simulink model "MPC_mobile_base_KIN_IPOPT_fast"  (R2018b)
settings: Solver=ode4  StartTime=0.0  StopTime=inf  FixedStep=Tsample  RelTol=1e-3
values from neighbouring files (symbols this model uses):
  initialize_starting_point = 1    [init_prova_vera1.mat]    (also in init_prova_vera3.mat; prova_vera1.mat = 0; prova_vera2.mat = 0)
  N = length(q)    [FK.m]    (also in FK_generation.m = size(DHTABLE,1); init_prova_vera1.mat = 10; init_prova_vera3.mat = 10; jacobian_MM.m)
  Np = 18    [init_prova_vera1.mat]    (also in init_prova_vera3.mat; initialization.m = Lf*2 + Lp*6; prova_vera1.mat; prova_vera2.mat)
  T = cell(N+1,1)    [FK.m]    (also in init_prova_vera1.mat = 0.5; init_prova_vera3.mat = 0.5; jacobian_MM.m; matlabultimo.mat = 0.5)
  Tsample = 0.01    [init_prova_vera1.mat]    (also in init_prova_vera3.mat; matlabultimo.mat; prova_vera1.mat; prova_vera2.mat)
  x0_val = [0 0 0 -5.2235 -1.0817 -2.0377 -0.3426 0.6332 1.3451 0.0238792670666 0.415141969475 1.22261425872 ... (18 elements, 18x1)]    [init_prova_vera1.mat]    (also in init_prova_vera3.mat; matlabultimo.mat = [0 0 0 2.943 -0.9502 1.3671 -2.8338 -2.9626 -0.0003 0.671714; prova_vera1.mat; prova_vera2.mat)
  xd = [0 0 0 0 0 0 0 0 0 0.0238792670666 0.415141969475 1.22261425872 ... (1458 elements, 18x81)]    [init_prova_vera1.mat]    (also in init_prova_vera3.mat; liveplot.m = evalin('base','xd'); matlabultimo.mat = [0 0 0 0 0 0 0 0 0 -0.528285242967 -0.106449885857 1.3372295; prova_vera1.mat)
undefined symbols (not defined in the file or in its folder): DiscIntNeverNeededParam
libraries: simulink x3
settings Model: Creator=francesco  LastModifiedBy=francesco
settings ModelReferenceCC: PropagateVarSize=Only when enabling

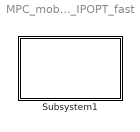
== system MPC_mobile_base_KIN_IPOPT_fast ==
  Subsystem1 : Subsystem  InitFcn=initialization

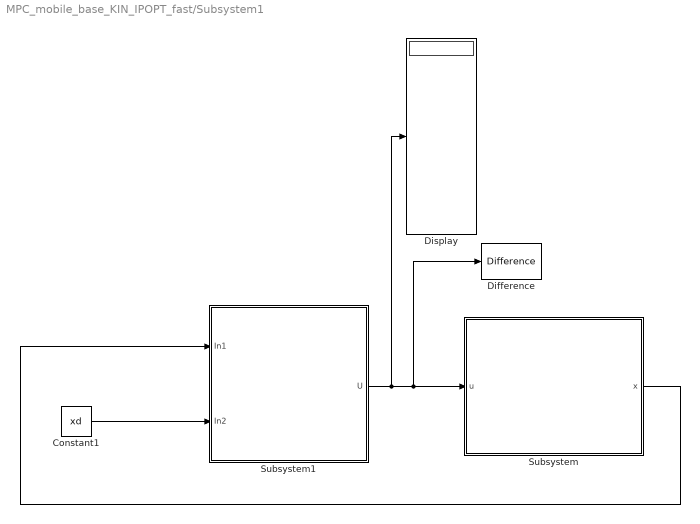
== system MPC_mobile_base_KIN_IPOPT_fast/Subsystem1 ==
  Constant1 : Constant  Value=xd
  Difference : simulink/Discrete/Difference  ICPrevInput=0.0  OutMin=[]  OutMax=[]  OutDataType=fixdt(1, 16)  OutScaling=2^-10  DoSatur=off
  Display : Display
  Subsystem : Subsystem
      mask Display: disp('{\bf\fontsize{10}KINEMATIC SYSTEM}', 'texmode','on');
  Subsystem1 : Subsystem
  wires:
  Subsystem1/1(U) -> Display/1, Difference/1, Subsystem/1(u)
  Constant1/1 -> Subsystem1/2(In2)
  Subsystem/1(x) -> Subsystem1/1(In1)

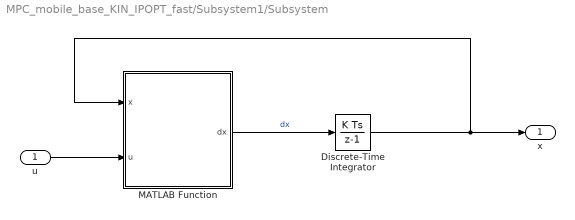
== system MPC_mobile_base_KIN_IPOPT_fast/Subsystem1/Subsystem ==
  u : Inport
  Discrete-Time Integrator : DiscreteIntegrator  InitialCondition=x0_val  SampleTime=Tsample  ICPrevOutput=DiscIntNeverNeededParam  ICPrevScaledInput=DiscIntNeverNeededParam
  MATLAB Function : MATLAB Function  TreatAsAtomicUnit=on
  x : Outport  SampleTime=Tsample
  wires:
  u/1 -> MATLAB Function/2(u)
  MATLAB Function/1(dx) -> Discrete-Time Integrator/1  "dx"
  Discrete-Time Integrator/1 -> MATLAB Function/1(x), x/1

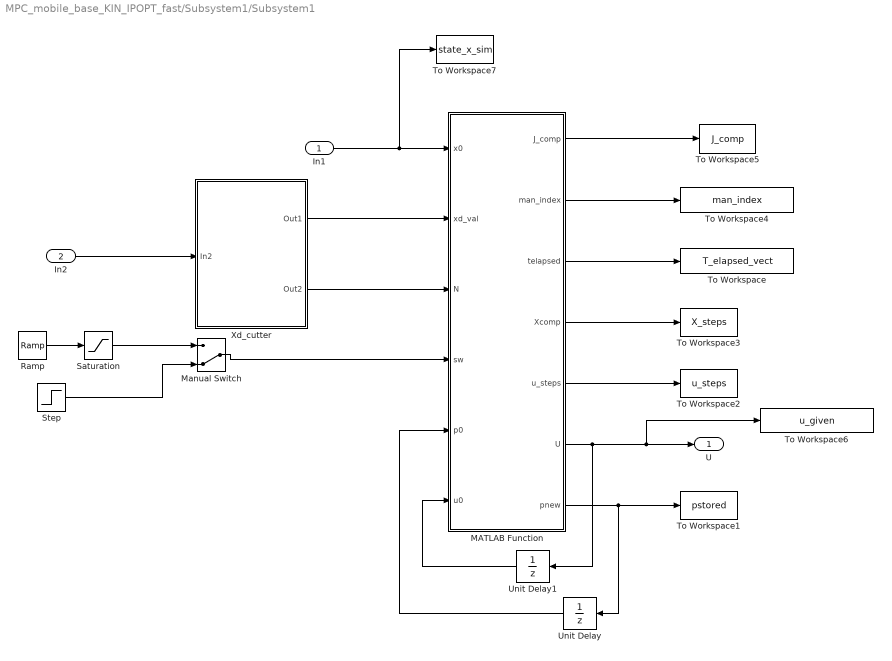
== system MPC_mobile_base_KIN_IPOPT_fast/Subsystem1/Subsystem1 ==
  In1 : Inport
  In2 : Inport  Port=2
  MATLAB Function : MATLAB Function  TreatAsAtomicUnit=on
  Manual Switch : ManualSwitch  CurrentSetting=0
  Ramp : simulink/Sources/Ramp  slope=1.5  start=15  InitialOutput=0
  Saturation : Saturate  UpperLimit=1
  Step : Step  Time=0  SampleTime=0
  To Workspace : ToWorkspace  VariableName=T_elapsed_vect  SampleTime=T
  To Workspace1 : ToWorkspace  VariableName=pstored  SampleTime=-1
  To Workspace2 : ToWorkspace  VariableName=u_steps  SaveFormat=Structure  SampleTime=-1
  To Workspace3 : ToWorkspace  VariableName=X_steps  SaveFormat=Structure  SampleTime=-1
  To Workspace4 : ToWorkspace  VariableName=man_index  SampleTime=T
  To Workspace5 : ToWorkspace  VariableName=J_comp  SampleTime=-1
  To Workspace6 : ToWorkspace  VariableName=u_given  SampleTime=T
  To Workspace7 : ToWorkspace  VariableName=state_x_sim  SampleTime=T
  Unit Delay : UnitDelay  InitialCondition=zeros(Np,1)  SampleTime=T
  Unit Delay1 : UnitDelay  InitialCondition=zeros(8,1)  SampleTime=T
  Xd_cutter : Subsystem
  U : Outport
  wires:
  MATLAB Function/7(pnew) -> To Workspace1/1, Unit Delay/1
  MATLAB Function/6(U) -> Unit Delay1/1, To Workspace6/1, U/1
  Unit Delay/1 -> MATLAB Function/5(p0)
  MATLAB Function/3(telapsed) -> To Workspace/1
  Unit Delay1/1 -> MATLAB Function/6(u0)
  MATLAB Function/5(u_steps) -> To Workspace2/1
  MATLAB Function/4(Xcomp) -> To Workspace3/1
  In2/1 -> Xd_cutter/1(In2)
  Xd_cutter/1(Out1) -> MATLAB Function/2(xd_val)
  Xd_cutter/2(Out2) -> MATLAB Function/3(N)
  Saturation/1 -> Manual Switch/1
  MATLAB Function/2(man_index) -> To Workspace4/1
  Ramp/1 -> Saturation/1
  Step/1 -> Manual Switch/2
  Manual Switch/1 -> MATLAB Function/4(sw)
  MATLAB Function/1(J_comp) -> To Workspace5/1
  In1/1 -> To Workspace7/1, MATLAB Function/1(x0)

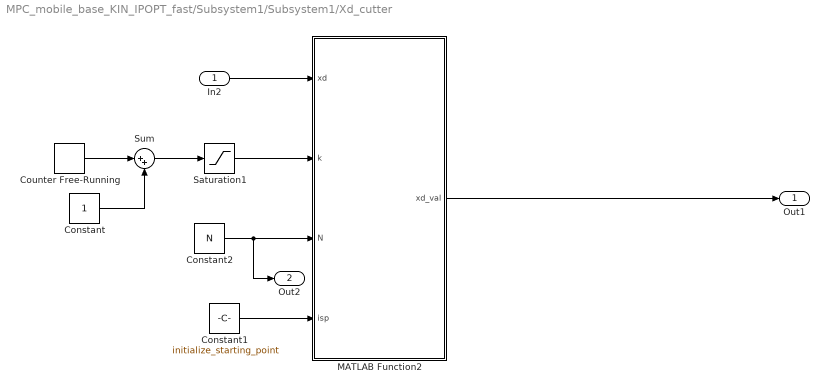
== system MPC_mobile_base_KIN_IPOPT_fast/Subsystem1/Subsystem1/Xd_cutter ==
  In2 : Inport
  Constant : Constant
  Constant1 : Constant  Value=initialize_starting_point
  Constant2 : Constant  Value=N
  Counter Free-Running : simulink/Sources/Counter Free-Running  NumBits=12  tsamp=T
  MATLAB Function2 : MATLAB Function  TreatAsAtomicUnit=on
  Saturation1 : Saturate  UpperLimit=size(xd,2)
  Sum : Sum  Inputs=|++
  Out1 : Outport
  Out2 : Outport  Port=2
  wires:
  Counter Free-Running/1 -> Sum/1
  Saturation1/1 -> MATLAB Function2/2(k)
  MATLAB Function2/1(xd_val) -> Out1/1
  Sum/1 -> Saturation1/1
  Constant/1 -> Sum/2
  Constant2/1 -> Out2/1, MATLAB Function2/3(N)
  In2/1 -> MATLAB Function2/1(xd)
  Constant1/1 -> MATLAB Function2/4(isp)

== matlab function MPC_mobile_base_KIN_IPOPT_fast/Subsystem1/Subsystem1/MATLAB Function ==
  settings: updateMethod=DISCRETE  sampleTime=T
  data: J_comp output; man_index output size=[1]; telapsed output; Xcomp output size=[19,N+1]; u_steps output size=[8,N]; U output; x0 input; pnew output size=[Np 1]; xd_val input; N input; sw input; p0 input; u0 input
function [J_comp,man_index,telapsed,Xcomp,u_steps,U,pnew] = fnc(x0,xd_val,N,sw,p0,u0)

coder.extrinsic('solver_NLP');
coder.extrinsic('evalin');
% Np = evalin('base','Np');

pnew=zeros(size(p0));

J_comp=zeros(1,6);

% INITIALIZING VARIABLES

telapsed=0;
u_steps=zeros(2,N);
U=zeros(8,1);
Xcomp=zeros(18,N);
man_index=0;

% SOLVING THE PROBLEM

[pnew, U, u_steps, Xcomp, telapsed, man, J_comp] = solver_NLP(xd_val,p0,x0,u0,sw);

man_index(1)=man;

end

== matlab function MPC_mobile_base_KIN_IPOPT_fast/Subsystem1/Subsystem1/Xd_cutter/MATLAB Function2 ==
  settings: updateMethod=DISCRETE  sampleTime=T
  data: xd input; k input; N input; xd_val output size=[18,N]; isp input
function xd_val = fcn(xd,k,N,isp)

    xd_val=zeros(18,N);

    if isp == 1
        xd_val=xd(:,1)*ones(1,N);
    else
        
        if size(xd,2)-k>N-1
        h=xd(:,k+1:k+N);

        else
        h=[xd(:,k+1:end) xd(:,end)*ones(1,N-(size(xd,2)-k))];

        end
    xd_val = h;

    end
end

== matlab function MPC_mobile_base_KIN_IPOPT_fast/Subsystem1/Subsystem/MATLAB Function ==
  settings: updateMethod=DISCRETE  sampleTime=Tsample
  data: x input; dx output; u input size=[8 1]
function dx = sys_dynamics(x,u)


G=[cos(x(3)) 0; sin(x(3)) 0; 0 1 ];

B = zeros(6,2);

dx = [   G                zeros(3,6)  ; ...
         zeros(6,2)       eye(6)      ; ...
         zeros(9,8)                   ]*u;

end
